simulink model "Xray"  (R2023b)
settings: Solver=VariableStepAuto  StartTime=0.0  StopTime=10.0  RelTol=1e-3
settings Model: Creator=user  LastModifiedBy=user

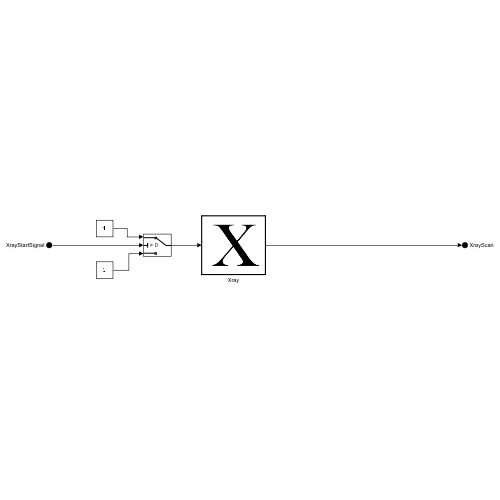
[thumbnail: Simulink's stored preview of the top-level diagram]
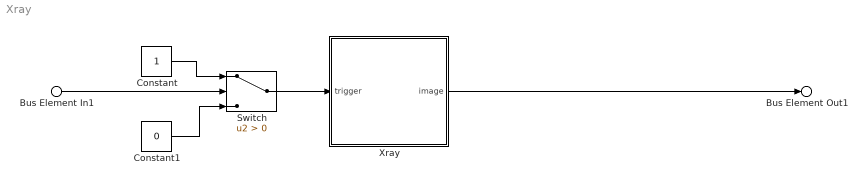
== system Xray ==
  Bus Element In1 : Inport  PortName=XrayStartSignal
  Constant : Constant
  Constant1 : Constant  Value=0
  Switch : Switch  Criteria=u2 > Threshold  SaturateOnIntegerOverflow=off  InputSameDT=off
  Xray : MATLAB Function  TreatAsAtomicUnit=on
  Bus Element Out1 : Outport  PortName=XrayScan
  wires:
  Switch/1 -> Xray/1(trigger)
  Constant/1 -> Switch/1
  Xray/1(image) -> Bus Element Out1/1
  Constant1/1 -> Switch/3
  Bus Element In1/1 -> Switch/2

== matlab function Xray/Xray ==
  data: trigger input; image output
function image = fcn(trigger)

u = 255*rand(200, 200, 2);


image = trigger;
